simulink model "stage5b_pi_anti_windup"  (R2024a)
settings: Solver=FixedStepDiscrete  StartTime=0.0  StopTime=3600  FixedStep=10  RelTol=1e-3
settings Model: Creator=Peter  LastModifiedBy=Peter

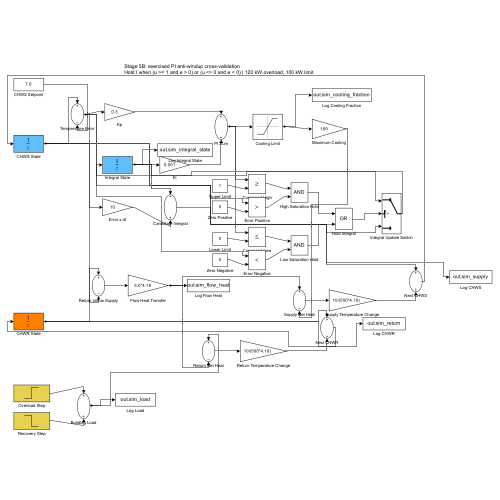
[thumbnail: Simulink's stored preview of the top-level diagram]
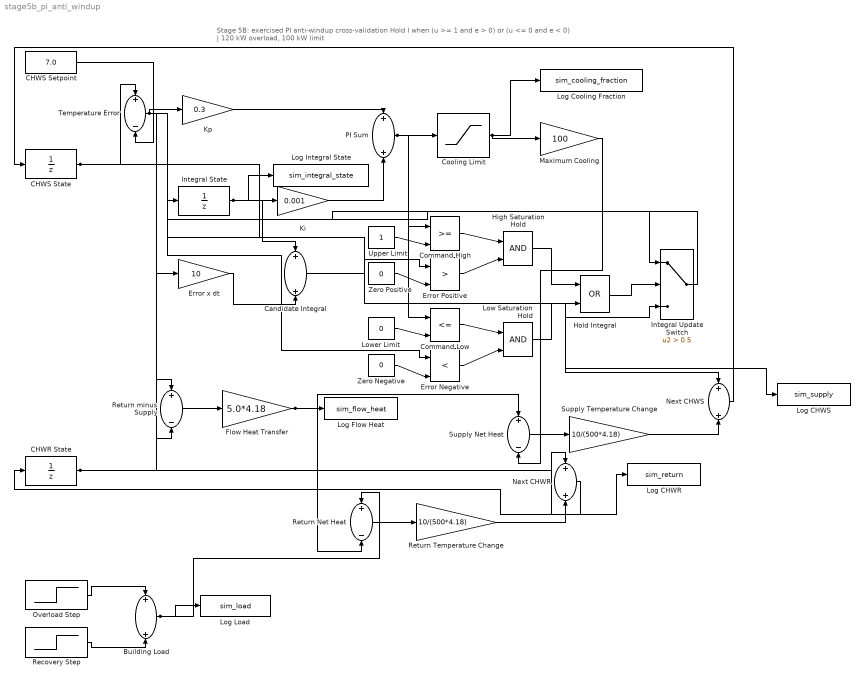
== system stage5b_pi_anti_windup ==
  note: Stage 5B: exercised PI anti-windup cross-validation
      | Hold I when (u >= 1 and e > 0) or (u <= 0 and e < 0) | 120 kW overload, 100 kW limit
  Building Load : Sum
  CHWR State : UnitDelay  InitialCondition=8.435406698564593  SampleTime=10  HasFrameUpgradeWarning=on
  CHWS Setpoint : Constant  Value=7.0
  CHWS State : UnitDelay  InitialCondition=7.0  SampleTime=10  HasFrameUpgradeWarning=on
  Candidate Integral : Sum
  Command High : RelationalOperator  OutDataTypeStr=boolean  RndMeth=Simplest  InputSameDT=off
  Command Low : RelationalOperator  Operator=<=  OutDataTypeStr=boolean  RndMeth=Simplest  InputSameDT=off
  Cooling Limit : Saturate  UpperLimit=1  LowerLimit=0
  Error Negative : RelationalOperator  Operator=<  OutDataTypeStr=boolean  RndMeth=Simplest  InputSameDT=off
  Error Positive : RelationalOperator  Operator=>  OutDataTypeStr=boolean  RndMeth=Simplest  InputSameDT=off
  Error x dt : Gain  Gain=10
  Flow Heat Transfer : Gain  Gain=5.0*4.18
  High Saturation Hold : Logic  AllPortsSameDT=off  OutDataTypeStr=boolean
  Hold Integral : Logic  Operator=OR  AllPortsSameDT=off  OutDataTypeStr=boolean
  Integral State : UnitDelay  InitialCondition=300  SampleTime=10  HasFrameUpgradeWarning=on
  Integral Update Switch : Switch  Criteria=u2 > Threshold  Threshold=0.5  SaturateOnIntegerOverflow=off  InputSameDT=off
  Ki : Gain  Gain=0.001
  Kp : Gain  Gain=0.3
  Log CHWR : ToWorkspace  VariableName=sim_return  SaveFormat=Timeseries  SampleTime=-1
  Log CHWS : ToWorkspace  VariableName=sim_supply  SaveFormat=Timeseries  SampleTime=-1
  Log Cooling Fraction : ToWorkspace  VariableName=sim_cooling_fraction  SaveFormat=Timeseries  SampleTime=-1
  Log Flow Heat : ToWorkspace  VariableName=sim_flow_heat  SaveFormat=Timeseries  SampleTime=-1
  Log Integral State : ToWorkspace  VariableName=sim_integral_state  SaveFormat=Timeseries  SampleTime=-1
  Log Load : ToWorkspace  VariableName=sim_load  SaveFormat=Timeseries  SampleTime=-1
  Low Saturation Hold : Logic  AllPortsSameDT=off  OutDataTypeStr=boolean
  Lower Limit : Constant  Value=0
  Maximum Cooling : Gain  Gain=100
  Next CHWR : Sum
  Next CHWS : Sum
  Overload Step : Step  Time=600  Before=30  After=120  SampleTime=10
  PI Sum : Sum
  Recovery Step : Step  Time=1200  After=-90  SampleTime=10
  Return Net Heat : Sum  Inputs=+-
  Return Temperature Change : Gain  Gain=10/(500*4.18)
  Return minus Supply : Sum  Inputs=+-
  Supply Net Heat : Sum  Inputs=+-
  Supply Temperature Change : Gain  Gain=10/(500*4.18)
  Temperature Error : Sum  Inputs=+-
  Upper Limit : Constant
  Zero Negative : Constant  Value=0
  Zero Positive : Constant  Value=0
  wires:
  CHWS State/1 -> Temperature Error/1, Return minus Supply/2, Next CHWS/1, Log CHWS/1
  CHWS Setpoint/1 -> Temperature Error/2
  Temperature Error/1 -> Kp/1, Error x dt/1, Error Positive/1, Error Negative/1
  Integral State/1 -> Ki/1, Candidate Integral/1, Integral Update Switch/1, Log Integral State/1
  Error x dt/1 -> Candidate Integral/2
  Kp/1 -> PI Sum/1
  Ki/1 -> PI Sum/2
  PI Sum/1 -> Cooling Limit/1, Command High/1, Command Low/1
  Cooling Limit/1 -> Maximum Cooling/1, Log Cooling Fraction/1
  Upper Limit/1 -> Command High/2
  Zero Positive/1 -> Error Positive/2
  Command High/1 -> High Saturation Hold/1
  Error Positive/1 -> High Saturation Hold/2
  Lower Limit/1 -> Command Low/2
  Zero Negative/1 -> Error Negative/2
  Command Low/1 -> Low Saturation Hold/1
  Error Negative/1 -> Low Saturation Hold/2
  High Saturation Hold/1 -> Hold Integral/1
  Low Saturation Hold/1 -> Hold Integral/2
  Hold Integral/1 -> Integral Update Switch/2
  Candidate Integral/1 -> Integral Update Switch/3
  Integral Update Switch/1 -> Integral State/1
  CHWR State/1 -> Return minus Supply/1, Next CHWR/1, Log CHWR/1
  Return minus Supply/1 -> Flow Heat Transfer/1
  Flow Heat Transfer/1 -> Supply Net Heat/1, Return Net Heat/2, Log Flow Heat/1
  Maximum Cooling/1 -> Supply Net Heat/2
  Supply Net Heat/1 -> Supply Temperature Change/1
  Supply Temperature Change/1 -> Next CHWS/2
  Next CHWS/1 -> CHWS State/1
  Overload Step/1 -> Building Load/1
  Recovery Step/1 -> Building Load/2
  Building Load/1 -> Return Net Heat/1, Log Load/1
  Return Net Heat/1 -> Return Temperature Change/1
  Return Temperature Change/1 -> Next CHWR/2
  Next CHWR/1 -> CHWR State/1
